simulink model "allmodes"  (Simulink 7.4)
settings: Solver=ode23tb  StartTime=0.0  StopTime=inf  MaxStep=1e-4  RelTol=1e-4
undefined symbols (not defined in the file): Ion, Lithium
libraries: powerlib x185, electricdrivelib x21, powerlib_extras x19, simulink x5
(part 4 of 7)

== system allmodes/vechicle units/vechicle-1 ==
  C1v1 : powerlib/Elements/Series RLC Branch  DialogController=POWERSYS.PowerSysDialog  PhysicalDomain=powersysdomain  SubClassName=unknown  LeftPortType=p1  RightPortType=p1  LConnTagsString=__new0  RConnTagsString=__new0  BranchType=C  Resistance=0.75  Inductance=1e-3  SetiL0=off  InitialCurrent=0  Capacitance=33e-5  Setx0=on  InitialVoltage=0  Measurements=Branch voltage and current
  Demux3 : Demux  Outputs=3
  Demux4 : Demux  Outputs=3
  IGBT20 : Subsystem
  IGBT21 : Subsystem
  L11v1 : powerlib/Elements/Series RLC Branch  DialogController=POWERSYS.PowerSysDialog  PhysicalDomain=powersysdomain  SubClassName=unknown  LeftPortType=p1  RightPortType=p1  LConnTagsString=__new0  RConnTagsString=__new0  BranchType=RL  Resistance=1e-3  Inductance=0.0033  SetiL0=off  InitialCurrent=0  Capacitance=1e-6  Setx0=off  InitialVoltage=0  Measurements=Branch voltage and current
  L22v1 : powerlib/Elements/Series RLC Branch  DialogController=POWERSYS.PowerSysDialog  PhysicalDomain=powersysdomain  SubClassName=unknown  LeftPortType=p1  RightPortType=p1  LConnTagsString=__new0  RConnTagsString=__new0  BranchType=RL  Resistance=1e-3  Inductance=1.2e-4  SetiL0=off  InitialCurrent=0  Capacitance=1e-6  Setx0=off  InitialVoltage=0  Measurements=Branch current
  Multimeter3 : powerlib/Measurements/Multimeter  SystemSampleTime=-1  PhasorSimulation=off  OutputType=Complex  sel=[5 58 59]  L=119  Gain=[1 1 1]  yselected={'Ub: vechicle units/vechicle-1/C1v1','Ib: vechicle units/vechicle-1/L11v1','Ib: vechicle units/vechicle-1/L22v1'};  PSBOutputType=1  PSBequivalent=0  AxesSetting=[0,0.1,-100,100]  Display=0  SavedBlockNames=-11
  v-1 : electricdrivelib/Extra Sources/Battery  DialogController=POWERSYS.PowerSysDialog  SystemSampleTime=-1  BatType=Lithium-Ion  ShowDetailedParameters=off  NomV=200  NomQ=30  SOC=10  PresetModel=on  MaxQ=30  FullV=232.7974  Dis_rate=13.0435  R=0.066667  Normal_OP=27.1304  expZone="[216.0772      1.473913]"  Dis_Char=off  current=[1.5 70]  Units=Ampere-hour  Batt_Tr=30
  +ve : PMIOPort  Port=1  Side=Left
  -ve : PMIOPort  Port=2  Side=Left
  tag scope: ISUIMv1=global, IbSUIMv1=global, Ibatv1=global, VbSUIMv1=global, VcSUIMv1=global, socv1=global
  wires:
  v-1/1 -> Demux4/1
  Demux4/1 -> [socv1]
  Demux4/2 -> [Ibatv1]
  Demux4/3 -> [VbSUIMv1]
  Multimeter3/1 -> Demux3/1
  Demux3/2 -> [ISUIMv1]
  Demux3/3 -> [IbSUIMv1]
  Demux3/1 -> [VcSUIMv1]
  connections:
  C1v1/LConn1 -- L22v1/LConn1 -- L11v1/RConn1
  -ve/RConn1 -- IGBT21/RConn2 -- v-1/LConn2 -- C1v1/RConn1
  IGBT20/RConn2 -- L11v1/LConn1 -- IGBT21/RConn1
  L22v1/RConn1 -- v-1/LConn1
  +ve/RConn1 -- IGBT20/RConn1

== system allmodes/vechicle units/vechicle-10 ==
  C1v10 : powerlib/Elements/Series RLC Branch  DialogController=POWERSYS.PowerSysDialog  PhysicalDomain=powersysdomain  SubClassName=unknown  LeftPortType=p1  RightPortType=p1  LConnTagsString=__new0  RConnTagsString=__new0  BranchType=C  Resistance=0.75  Inductance=1e-3  SetiL0=off  InitialCurrent=0  Capacitance=33e-6  Setx0=on  InitialVoltage=0  Measurements=Branch voltage and current
  Demux3 : Demux  Outputs=3
  Demux4 : Demux  Outputs=3
  IGBT20 : Subsystem
  IGBT21 : Subsystem
  L11v10 : powerlib/Elements/Series RLC Branch  DialogController=POWERSYS.PowerSysDialog  PhysicalDomain=powersysdomain  SubClassName=unknown  LeftPortType=p1  RightPortType=p1  LConnTagsString=__new0  RConnTagsString=__new0  BranchType=RL  Resistance=1e-3  Inductance=0.0033  SetiL0=off  InitialCurrent=0  Capacitance=1e-6  Setx0=off  InitialVoltage=0  Measurements=Branch voltage and current
  L22v10 : powerlib/Elements/Series RLC Branch  DialogController=POWERSYS.PowerSysDialog  PhysicalDomain=powersysdomain  SubClassName=unknown  LeftPortType=p1  RightPortType=p1  LConnTagsString=__new0  RConnTagsString=__new0  BranchType=RL  Resistance=0.001  Inductance=1.2e-4  SetiL0=off  InitialCurrent=0  Capacitance=1e-6  Setx0=off  InitialVoltage=0  Measurements=Branch current
  Multimeter3 : powerlib/Measurements/Multimeter  SystemSampleTime=-1  PhasorSimulation=off  OutputType=Complex  sel=[7 61 62]  L=119  Gain=[1 1 1]  yselected={'Ub: vechicle units/vechicle-10/C1v10','Ib: vechicle units/vechicle-10/L11v10','Ib: vechicle units/vechicle-10/L22v10'};  PSBOutputType=1  PSBequivalent=0  AxesSetting=[0,0.1,-100,100]  Display=0  SavedBlockNames=-11
  v-10 : electricdrivelib/Extra Sources/Battery  DialogController=POWERSYS.PowerSysDialog  SystemSampleTime=-1  BatType=Lithium-Ion  ShowDetailedParameters=off  NomV=200  NomQ=30  SOC=50  PresetModel=on  MaxQ=30  FullV=232.7974  Dis_rate=13.0435  R=0.066667  Normal_OP=27.1304  expZone="[216.0772      1.473913]"  Dis_Char=off  current=[1.5 70]  Units=Ampere-hour  Batt_Tr=30
  +ve : PMIOPort  Port=1  Side=Left
  -ve : PMIOPort  Port=2  Side=Left
  tag scope: ISUIMv10=global, IbSUIMv10=global, Ibatv10=global, VbSUIMv10=global, VcSUIMv10=global, socv10=global
  wires:
  Demux3/1 -> [VcSUIMv10]
  Demux3/3 -> [IbSUIMv10]
  Demux3/2 -> [ISUIMv10]
  Multimeter3/1 -> Demux3/1
  Demux4/3 -> [VbSUIMv10]
  Demux4/2 -> [Ibatv10]
  Demux4/1 -> [socv10]
  v-10/1 -> Demux4/1
  connections:
  +ve/RConn1 -- IGBT20/RConn1
  L22v10/RConn1 -- v-10/LConn1
  IGBT21/RConn1 -- IGBT20/RConn2 -- L11v10/LConn1
  IGBT21/RConn2 -- -ve/RConn1 -- C1v10/RConn1 -- v-10/LConn2
  L11v10/RConn1 -- L22v10/LConn1 -- C1v10/LConn1

== system allmodes/vechicle units/vechicle-11 ==
  C1v11 : powerlib/Elements/Series RLC Branch  DialogController=POWERSYS.PowerSysDialog  PhysicalDomain=powersysdomain  SubClassName=unknown  LeftPortType=p1  RightPortType=p1  LConnTagsString=__new0  RConnTagsString=__new0  BranchType=C  Resistance=0.75  Inductance=1e-3  SetiL0=off  InitialCurrent=0  Capacitance=33e-6  Setx0=on  InitialVoltage=0  Measurements=Branch voltage and current
  Demux3 : Demux  Outputs=3
  Demux4 : Demux  Outputs=3
  IGBT20 : Subsystem
  IGBT21 : Subsystem
  L11v11 : powerlib/Elements/Series RLC Branch  DialogController=POWERSYS.PowerSysDialog  PhysicalDomain=powersysdomain  SubClassName=unknown  LeftPortType=p1  RightPortType=p1  LConnTagsString=__new0  RConnTagsString=__new0  BranchType=RL  Resistance=0.001  Inductance=0.0033  SetiL0=off  InitialCurrent=0  Capacitance=1e-6  Setx0=off  InitialVoltage=0  Measurements=Branch voltage and current
  L22v11 : powerlib/Elements/Series RLC Branch  DialogController=POWERSYS.PowerSysDialog  PhysicalDomain=powersysdomain  SubClassName=unknown  LeftPortType=p1  RightPortType=p1  LConnTagsString=__new0  RConnTagsString=__new0  BranchType=RL  Resistance=0.001  Inductance=1.2e-4  SetiL0=off  InitialCurrent=0  Capacitance=1e-6  Setx0=off  InitialVoltage=0  Measurements=Branch current
  Multimeter3 : powerlib/Measurements/Multimeter  SystemSampleTime=-1  PhasorSimulation=off  OutputType=Complex  sel=[9 64 65]  L=119  Gain=[1 1 1]  yselected={'Ub: vechicle units/vechicle-11/C1v11','Ib: vechicle units/vechicle-11/L11v11','Ib: vechicle units/vechicle-11/L22v11'};  PSBOutputType=1  PSBequivalent=0  AxesSetting=[0,0.1,-100,100]  Display=0  SavedBlockNames=-11
  v-11 : electricdrivelib/Extra Sources/Battery  DialogController=POWERSYS.PowerSysDialog  SystemSampleTime=-1  BatType=Lithium-Ion  ShowDetailedParameters=off  NomV=200  NomQ=30  SOC=50  PresetModel=on  MaxQ=30  FullV=232.7974  Dis_rate=13.0435  R=0.066667  Normal_OP=27.1304  expZone="[216.0772      1.473913]"  Dis_Char=off  current=[1.5 70]  Units=Ampere-hour  Batt_Tr=30
  +ve : PMIOPort  Port=1  Side=Left
  -ve : PMIOPort  Port=2  Side=Left
  tag scope: ISUIMv11=global, IbSUIMv11=global, Ibatv11=global, VbSUIMv11=global, VcSUIMv11=global, socv11=global
  wires:
  v-11/1 -> Demux4/1
  Demux4/1 -> [socv11]
  Demux4/2 -> [Ibatv11]
  Demux4/3 -> [VbSUIMv11]
  Multimeter3/1 -> Demux3/1
  Demux3/2 -> [ISUIMv11]
  Demux3/3 -> [IbSUIMv11]
  Demux3/1 -> [VcSUIMv11]
  connections:
  C1v11/LConn1 -- L22v11/LConn1 -- L11v11/RConn1
  v-11/LConn2 -- C1v11/RConn1 -- -ve/RConn1 -- IGBT21/RConn2
  L11v11/LConn1 -- IGBT20/RConn2 -- IGBT21/RConn1
  L22v11/RConn1 -- v-11/LConn1
  +ve/RConn1 -- IGBT20/RConn1

== system allmodes/vechicle units/vechicle-12 ==
  C1v12 : powerlib/Elements/Series RLC Branch  DialogController=POWERSYS.PowerSysDialog  PhysicalDomain=powersysdomain  SubClassName=unknown  LeftPortType=p1  RightPortType=p1  LConnTagsString=__new0  RConnTagsString=__new0  BranchType=C  Resistance=0.75  Inductance=1e-3  SetiL0=off  InitialCurrent=0  Capacitance=33e-6  Setx0=on  InitialVoltage=0  Measurements=Branch voltage and current
  Demux3 : Demux  Outputs=3
  Demux4 : Demux  Outputs=3
  IGBT20 : Subsystem
  IGBT21 : Subsystem
  L11v12 : powerlib/Elements/Series RLC Branch  DialogController=POWERSYS.PowerSysDialog  PhysicalDomain=powersysdomain  SubClassName=unknown  LeftPortType=p1  RightPortType=p1  LConnTagsString=__new0  RConnTagsString=__new0  BranchType=RL  Resistance=0.001  Inductance=0.0033  SetiL0=off  InitialCurrent=0  Capacitance=1e-6  Setx0=off  InitialVoltage=0  Measurements=Branch voltage and current
  L22v12 : powerlib/Elements/Series RLC Branch  DialogController=POWERSYS.PowerSysDialog  PhysicalDomain=powersysdomain  SubClassName=unknown  LeftPortType=p1  RightPortType=p1  LConnTagsString=__new0  RConnTagsString=__new0  BranchType=RL  Resistance=0.001  Inductance=1.2e-4  SetiL0=off  InitialCurrent=0  Capacitance=1e-6  Setx0=off  InitialVoltage=0  Measurements=Branch current
  Multimeter3 : powerlib/Measurements/Multimeter  SystemSampleTime=-1  PhasorSimulation=off  OutputType=Complex  sel=[11 67 68]  L=119  Gain=[1 1 1]  yselected={'Ub: vechicle units/vechicle-12/C1v12','Ib: vechicle units/vechicle-12/L11v12','Ib: vechicle units/vechicle-12/L22v12'};  PSBOutputType=1  PSBequivalent=0  AxesSetting=[0,0.1,-100,100]  Display=0  SavedBlockNames=-11
  v-12 : electricdrivelib/Extra Sources/Battery  DialogController=POWERSYS.PowerSysDialog  SystemSampleTime=-1  BatType=Lithium-Ion  ShowDetailedParameters=off  NomV=200  NomQ=30  SOC=50  PresetModel=on  MaxQ=30  FullV=232.7974  Dis_rate=13.0435  R=0.066667  Normal_OP=27.1304  expZone="[216.0772      1.473913]"  Dis_Char=off  current=[1.5 70]  Units=Ampere-hour  Batt_Tr=30
  +ve : PMIOPort  Port=1  Side=Left
  -ve : PMIOPort  Port=2  Side=Left
  tag scope: ISUIMv12=global, IbSUIMv12=global, Ibatv12=global, VbSUIMv12=global, VcSUIMv12=global, socv12=global
  wires:
  Demux3/1 -> [VcSUIMv12]
  Demux3/3 -> [IbSUIMv12]
  Demux3/2 -> [ISUIMv12]
  Multimeter3/1 -> Demux3/1
  Demux4/3 -> [VbSUIMv12]
  Demux4/2 -> [Ibatv12]
  Demux4/1 -> [socv12]
  v-12/1 -> Demux4/1
  connections:
  +ve/RConn1 -- IGBT20/RConn1
  L22v12/RConn1 -- v-12/LConn1
  IGBT21/RConn1 -- IGBT20/RConn2 -- L11v12/LConn1
  IGBT21/RConn2 -- -ve/RConn1 -- C1v12/RConn1 -- v-12/LConn2
  L11v12/RConn1 -- L22v12/LConn1 -- C1v12/LConn1

== system allmodes/vechicle units/vechicle-13 ==
  C1v13 : powerlib/Elements/Series RLC Branch  DialogController=POWERSYS.PowerSysDialog  PhysicalDomain=powersysdomain  SubClassName=unknown  LeftPortType=p1  RightPortType=p1  LConnTagsString=__new0  RConnTagsString=__new0  BranchType=C  Resistance=0.75  Inductance=1e-3  SetiL0=off  InitialCurrent=0  Capacitance=33e-6  Setx0=on  InitialVoltage=0  Measurements=Branch voltage and current
  Demux3 : Demux  Outputs=3
  Demux4 : Demux  Outputs=3
  IGBT20 : Subsystem
  IGBT21 : Subsystem
  L11v13 : powerlib/Elements/Series RLC Branch  DialogController=POWERSYS.PowerSysDialog  PhysicalDomain=powersysdomain  SubClassName=unknown  LeftPortType=p1  RightPortType=p1  LConnTagsString=__new0  RConnTagsString=__new0  BranchType=RL  Resistance=0.001  Inductance=0.0033  SetiL0=off  InitialCurrent=0  Capacitance=1e-6  Setx0=off  InitialVoltage=0  Measurements=Branch voltage and current
  L22v13 : powerlib/Elements/Series RLC Branch  DialogController=POWERSYS.PowerSysDialog  PhysicalDomain=powersysdomain  SubClassName=unknown  LeftPortType=p1  RightPortType=p1  LConnTagsString=__new0  RConnTagsString=__new0  BranchType=RL  Resistance=0.001  Inductance=1.2e-4  SetiL0=off  InitialCurrent=0  Capacitance=1e-6  Setx0=off  InitialVoltage=0  Measurements=Branch current
  Multimeter3 : powerlib/Measurements/Multimeter  SystemSampleTime=-1  PhasorSimulation=off  OutputType=Complex  sel=[13 70 71]  L=119  Gain=[1 1 1]  yselected={'Ub: vechicle units/vechicle-13/C1v13','Ib: vechicle units/vechicle-13/L11v13','Ib: vechicle units/vechicle-13/L22v13'};  PSBOutputType=1  PSBequivalent=0  AxesSetting=[0,0.1,-100,100]  Display=0  SavedBlockNames=-11
  v-13 : electricdrivelib/Extra Sources/Battery  DialogController=POWERSYS.PowerSysDialog  SystemSampleTime=-1  BatType=Lithium-Ion  ShowDetailedParameters=off  NomV=200  NomQ=30  SOC=50  PresetModel=on  MaxQ=30  FullV=232.7974  Dis_rate=13.0435  R=0.066667  Normal_OP=27.1304  expZone="[216.0772      1.473913]"  Dis_Char=off  current=[1.5 70]  Units=Ampere-hour  Batt_Tr=30
  +ve : PMIOPort  Port=1  Side=Left
  -ve : PMIOPort  Port=2  Side=Left
  tag scope: ISUIMv13=global, IbSUIMv13=global, Ibatv13=global, VbSUIMv13=global, VcSUIMv13=global, socv13=global
  wires:
  v-13/1 -> Demux4/1
  Demux4/1 -> [socv13]
  Demux4/2 -> [Ibatv13]
  Demux4/3 -> [VbSUIMv13]
  Multimeter3/1 -> Demux3/1
  Demux3/2 -> [ISUIMv13]
  Demux3/3 -> [IbSUIMv13]
  Demux3/1 -> [VcSUIMv13]
  connections:
  C1v13/LConn1 -- L22v13/LConn1 -- L11v13/RConn1
  v-13/LConn2 -- C1v13/RConn1 -- -ve/RConn1 -- IGBT21/RConn2
  L11v13/LConn1 -- IGBT20/RConn2 -- IGBT21/RConn1
  L22v13/RConn1 -- v-13/LConn1
  +ve/RConn1 -- IGBT20/RConn1

== system allmodes/vechicle units/vechicle-14 ==
  C1v14 : powerlib/Elements/Series RLC Branch  DialogController=POWERSYS.PowerSysDialog  PhysicalDomain=powersysdomain  SubClassName=unknown  LeftPortType=p1  RightPortType=p1  LConnTagsString=__new0  RConnTagsString=__new0  BranchType=C  Resistance=0.75  Inductance=1e-3  SetiL0=off  InitialCurrent=0  Capacitance=33e-6  Setx0=on  InitialVoltage=0  Measurements=Branch voltage and current
  Demux3 : Demux  Outputs=3
  Demux4 : Demux  Outputs=3
  IGBT20 : Subsystem
  IGBT21 : Subsystem
  L11v14 : powerlib/Elements/Series RLC Branch  DialogController=POWERSYS.PowerSysDialog  PhysicalDomain=powersysdomain  SubClassName=unknown  LeftPortType=p1  RightPortType=p1  LConnTagsString=__new0  RConnTagsString=__new0  BranchType=RL  Resistance=0.001  Inductance=0.0033  SetiL0=off  InitialCurrent=0  Capacitance=1e-6  Setx0=off  InitialVoltage=0  Measurements=Branch voltage and current
  L22v14 : powerlib/Elements/Series RLC Branch  DialogController=POWERSYS.PowerSysDialog  PhysicalDomain=powersysdomain  SubClassName=unknown  LeftPortType=p1  RightPortType=p1  LConnTagsString=__new0  RConnTagsString=__new0  BranchType=RL  Resistance=0.001  Inductance=1.2e-4  SetiL0=off  InitialCurrent=0  Capacitance=1e-6  Setx0=off  InitialVoltage=0  Measurements=Branch current
  Multimeter3 : powerlib/Measurements/Multimeter  SystemSampleTime=-1  PhasorSimulation=off  OutputType=Complex  sel=[15 73 74]  L=119  Gain=[1 1 1]  yselected={'Ub: vechicle units/vechicle-14/C1v14','Ib: vechicle units/vechicle-14/L11v14','Ib: vechicle units/vechicle-14/L22v14'};  PSBOutputType=1  PSBequivalent=0  AxesSetting=[0,0.1,-100,100]  Display=0  SavedBlockNames=-11
  v-14 : electricdrivelib/Extra Sources/Battery  DialogController=POWERSYS.PowerSysDialog  SystemSampleTime=-1  BatType=Lithium-Ion  ShowDetailedParameters=off  NomV=200  NomQ=30  SOC=50  PresetModel=on  MaxQ=30  FullV=232.7974  Dis_rate=13.0435  R=0.066667  Normal_OP=27.1304  expZone="[216.0772      1.473913]"  Dis_Char=off  current=[1.5 70]  Units=Ampere-hour  Batt_Tr=30
  +ve : PMIOPort  Port=1  Side=Left
  -ve : PMIOPort  Port=2  Side=Left
  tag scope: ISUIMv14=global, IbSUIMv14=global, Ibatv14=global, VbSUIMv14=global, VcSUIMv14=global, socv14=global
  wires:
  Demux3/1 -> [VcSUIMv14]
  Demux3/3 -> [IbSUIMv14]
  Demux3/2 -> [ISUIMv14]
  Multimeter3/1 -> Demux3/1
  Demux4/3 -> [VbSUIMv14]
  Demux4/2 -> [Ibatv14]
  Demux4/1 -> [socv14]
  v-14/1 -> Demux4/1
  connections:
  +ve/RConn1 -- IGBT20/RConn1
  L22v14/RConn1 -- v-14/LConn1
  IGBT21/RConn1 -- IGBT20/RConn2 -- L11v14/LConn1
  IGBT21/RConn2 -- -ve/RConn1 -- C1v14/RConn1 -- v-14/LConn2
  L11v14/RConn1 -- L22v14/LConn1 -- C1v14/LConn1

== system allmodes/vechicle units/vechicle-15 ==
  C1v15 : powerlib/Elements/Series RLC Branch  DialogController=POWERSYS.PowerSysDialog  PhysicalDomain=powersysdomain  SubClassName=unknown  LeftPortType=p1  RightPortType=p1  LConnTagsString=__new0  RConnTagsString=__new0  BranchType=C  Resistance=0.75  Inductance=1e-3  SetiL0=off  InitialCurrent=0  Capacitance=33e-6  Setx0=on  InitialVoltage=0  Measurements=Branch voltage and current
  Demux3 : Demux  Outputs=3
  Demux4 : Demux  Outputs=3
  IGBT20 : Subsystem
  IGBT21 : Subsystem
  L11v15 : powerlib/Elements/Series RLC Branch  DialogController=POWERSYS.PowerSysDialog  PhysicalDomain=powersysdomain  SubClassName=unknown  LeftPortType=p1  RightPortType=p1  LConnTagsString=__new0  RConnTagsString=__new0  BranchType=RL  Resistance=0.001  Inductance=0.0033  SetiL0=off  InitialCurrent=0  Capacitance=1e-6  Setx0=off  InitialVoltage=0  Measurements=Branch voltage and current
  L22v15 : powerlib/Elements/Series RLC Branch  DialogController=POWERSYS.PowerSysDialog  PhysicalDomain=powersysdomain  SubClassName=unknown  LeftPortType=p1  RightPortType=p1  LConnTagsString=__new0  RConnTagsString=__new0  BranchType=RL  Resistance=0.001  Inductance=1.21e-4  SetiL0=off  InitialCurrent=0  Capacitance=1e-6  Setx0=off  InitialVoltage=0  Measurements=Branch current
  Multimeter3 : powerlib/Measurements/Multimeter  SystemSampleTime=-1  PhasorSimulation=off  OutputType=Complex  sel=[17 76 77]  L=119  Gain=[1 1 1]  yselected={'Ub: vechicle units/vechicle-15/C1v15','Ib: vechicle units/vechicle-15/L11v15','Ib: vechicle units/vechicle-15/L22v15'};  PSBOutputType=1  PSBequivalent=0  AxesSetting=[0,0.1,-100,100]  Display=0  SavedBlockNames=-11
  v-15 : electricdrivelib/Extra Sources/Battery  DialogController=POWERSYS.PowerSysDialog  SystemSampleTime=-1  BatType=Lithium-Ion  ShowDetailedParameters=off  NomV=200  NomQ=30  SOC=50  PresetModel=on  MaxQ=30  FullV=232.7974  Dis_rate=13.0435  R=0.066667  Normal_OP=27.1304  expZone="[216.0772      1.473913]"  Dis_Char=off  current=[1.5 70]  Units=Ampere-hour  Batt_Tr=30
  +ve : PMIOPort  Port=1  Side=Left
  -ve : PMIOPort  Port=2  Side=Left
  tag scope: ISUIMv15=global, IbSUIMv15=global, Ibatv15=global, VbSUIMv15=global, VcSUIMv15=global, socv15=global
  wires:
  v-15/1 -> Demux4/1
  Demux4/1 -> [socv15]
  Demux4/2 -> [Ibatv15]
  Demux4/3 -> [VbSUIMv15]
  Multimeter3/1 -> Demux3/1
  Demux3/2 -> [ISUIMv15]
  Demux3/3 -> [IbSUIMv15]
  Demux3/1 -> [VcSUIMv15]
  connections:
  C1v15/LConn1 -- L22v15/LConn1 -- L11v15/RConn1
  v-15/LConn2 -- C1v15/RConn1 -- -ve/RConn1 -- IGBT21/RConn2
  L11v15/LConn1 -- IGBT20/RConn2 -- IGBT21/RConn1
  L22v15/RConn1 -- v-15/LConn1
  +ve/RConn1 -- IGBT20/RConn1

== system allmodes/vechicle units/vechicle-16 ==
  C1v16 : powerlib/Elements/Series RLC Branch  DialogController=POWERSYS.PowerSysDialog  PhysicalDomain=powersysdomain  SubClassName=unknown  LeftPortType=p1  RightPortType=p1  LConnTagsString=__new0  RConnTagsString=__new0  BranchType=C  Resistance=0.75  Inductance=1e-3  SetiL0=off  InitialCurrent=0  Capacitance=33e-6  Setx0=on  InitialVoltage=0  Measurements=Branch voltage and current
  Demux3 : Demux  Outputs=3
  Demux4 : Demux  Outputs=3
  IGBT20 : Subsystem
  IGBT21 : Subsystem
  L11v16 : powerlib/Elements/Series RLC Branch  DialogController=POWERSYS.PowerSysDialog  PhysicalDomain=powersysdomain  SubClassName=unknown  LeftPortType=p1  RightPortType=p1  LConnTagsString=__new0  RConnTagsString=__new0  BranchType=RL  Resistance=0.001  Inductance=0.0033  SetiL0=off  InitialCurrent=0  Capacitance=1e-6  Setx0=off  InitialVoltage=0  Measurements=Branch voltage and current
  L22v16 : powerlib/Elements/Series RLC Branch  DialogController=POWERSYS.PowerSysDialog  PhysicalDomain=powersysdomain  SubClassName=unknown  LeftPortType=p1  RightPortType=p1  LConnTagsString=__new0  RConnTagsString=__new0  BranchType=RL  Resistance=0.001  Inductance=1.2e-4  SetiL0=off  InitialCurrent=0  Capacitance=1e-6  Setx0=off  InitialVoltage=0  Measurements=Branch current
  Multimeter3 : powerlib/Measurements/Multimeter  SystemSampleTime=-1  PhasorSimulation=off  OutputType=Complex  sel=[19 79 80]  L=119  Gain=[1 1 1]  yselected={'Ub: vechicle units/vechicle-16/C1v16','Ib: vechicle units/vechicle-16/L11v16','Ib: vechicle units/vechicle-16/L22v16'};  PSBOutputType=1  PSBequivalent=0  AxesSetting=[0,0.1,-100,100]  Display=0  SavedBlockNames=-11
  v-16 : electricdrivelib/Extra Sources/Battery  DialogController=POWERSYS.PowerSysDialog  SystemSampleTime=-1  BatType=Lithium-Ion  ShowDetailedParameters=off  NomV=200  NomQ=30  SOC=50  PresetModel=on  MaxQ=30  FullV=232.7974  Dis_rate=13.0435  R=0.066667  Normal_OP=27.1304  expZone="[216.0772      1.473913]"  Dis_Char=off  current=[1.5 70]  Units=Ampere-hour  Batt_Tr=30
  +ve : PMIOPort  Port=1  Side=Left
  -ve : PMIOPort  Port=2  Side=Left
  tag scope: ISUIMv16=global, IbSUIMv16=global, Ibatv16=global, VbSUIMv16=global, VcSUIMv16=global, socv16=global
  wires:
  Demux3/1 -> [VcSUIMv16]
  Demux3/3 -> [IbSUIMv16]
  Demux3/2 -> [ISUIMv16]
  Multimeter3/1 -> Demux3/1
  Demux4/3 -> [VbSUIMv16]
  Demux4/2 -> [Ibatv16]
  Demux4/1 -> [socv16]
  v-16/1 -> Demux4/1
  connections:
  +ve/RConn1 -- IGBT20/RConn1
  L22v16/RConn1 -- v-16/LConn1
  IGBT21/RConn1 -- IGBT20/RConn2 -- L11v16/LConn1
  IGBT21/RConn2 -- -ve/RConn1 -- C1v16/RConn1 -- v-16/LConn2
  L11v16/RConn1 -- L22v16/LConn1 -- C1v16/LConn1

== system allmodes/vechicle units/vechicle-17 ==
  C1v17 : powerlib/Elements/Series RLC Branch  DialogController=POWERSYS.PowerSysDialog  PhysicalDomain=powersysdomain  SubClassName=unknown  LeftPortType=p1  RightPortType=p1  LConnTagsString=__new0  RConnTagsString=__new0  BranchType=C  Resistance=0.75  Inductance=1e-3  SetiL0=off  InitialCurrent=0  Capacitance=33e-6  Setx0=on  InitialVoltage=0  Measurements=Branch voltage and current
  Demux3 : Demux  Outputs=3
  Demux4 : Demux  Outputs=3
  IGBT20 : Subsystem
  IGBT21 : Subsystem
  L11v17 : powerlib/Elements/Series RLC Branch  DialogController=POWERSYS.PowerSysDialog  PhysicalDomain=powersysdomain  SubClassName=unknown  LeftPortType=p1  RightPortType=p1  LConnTagsString=__new0  RConnTagsString=__new0  BranchType=RL  Resistance=0.001  Inductance=0.0033  SetiL0=off  InitialCurrent=0  Capacitance=1e-6  Setx0=off  InitialVoltage=0  Measurements=Branch voltage and current
  L22v17 : powerlib/Elements/Series RLC Branch  DialogController=POWERSYS.PowerSysDialog  PhysicalDomain=powersysdomain  SubClassName=unknown  LeftPortType=p1  RightPortType=p1  LConnTagsString=__new0  RConnTagsString=__new0  BranchType=RL  Resistance=0.001  Inductance=1.2e-4  SetiL0=off  InitialCurrent=0  Capacitance=1e-6  Setx0=off  InitialVoltage=0  Measurements=Branch current
  Multimeter3 : powerlib/Measurements/Multimeter  SystemSampleTime=-1  PhasorSimulation=off  OutputType=Complex  sel=[21 82 83]  L=119  Gain=[1 1 1]  yselected={'Ub: vechicle units/vechicle-17/C1v17','Ib: vechicle units/vechicle-17/L11v17','Ib: vechicle units/vechicle-17/L22v17'};  PSBOutputType=1  PSBequivalent=0  AxesSetting=[0,0.1,-100,100]  Display=0  SavedBlockNames=-11
  v-17 : electricdrivelib/Extra Sources/Battery  DialogController=POWERSYS.PowerSysDialog  SystemSampleTime=-1  BatType=Lithium-Ion  ShowDetailedParameters=off  NomV=200  NomQ=30  SOC=50  PresetModel=on  MaxQ=30  FullV=232.7974  Dis_rate=13.0435  R=0.066667  Normal_OP=27.1304  expZone="[216.0772      1.473913]"  Dis_Char=off  current=[1.5 70]  Units=Ampere-hour  Batt_Tr=30
  +ve : PMIOPort  Port=1  Side=Left
  -ve : PMIOPort  Port=2  Side=Left
  tag scope: ISUIMv17=global, IbSUIMv17=global, Ibatv17=global, VbSUIMv17=global, VcSUIMv17=global, socv17=global
  wires:
  v-17/1 -> Demux4/1
  Demux4/1 -> [socv17]
  Demux4/2 -> [Ibatv17]
  Demux4/3 -> [VbSUIMv17]
  Multimeter3/1 -> Demux3/1
  Demux3/2 -> [ISUIMv17]
  Demux3/3 -> [IbSUIMv17]
  Demux3/1 -> [VcSUIMv17]
  connections:
  C1v17/LConn1 -- L22v17/LConn1 -- L11v17/RConn1
  v-17/LConn2 -- C1v17/RConn1 -- -ve/RConn1 -- IGBT21/RConn2
  L11v17/LConn1 -- IGBT20/RConn2 -- IGBT21/RConn1
  L22v17/RConn1 -- v-17/LConn1
  +ve/RConn1 -- IGBT20/RConn1

== system allmodes/vechicle units/vechicle-18 ==
  C1v18 : powerlib/Elements/Series RLC Branch  DialogController=POWERSYS.PowerSysDialog  PhysicalDomain=powersysdomain  SubClassName=unknown  LeftPortType=p1  RightPortType=p1  LConnTagsString=__new0  RConnTagsString=__new0  BranchType=C  Resistance=0.75  Inductance=1e-3  SetiL0=off  InitialCurrent=0  Capacitance=33e-6  Setx0=on  InitialVoltage=0  Measurements=Branch voltage and current
  Demux3 : Demux  Outputs=3
  Demux4 : Demux  Outputs=3
  IGBT20 : Subsystem
  IGBT21 : Subsystem
  L11v18 : powerlib/Elements/Series RLC Branch  DialogController=POWERSYS.PowerSysDialog  PhysicalDomain=powersysdomain  SubClassName=unknown  LeftPortType=p1  RightPortType=p1  LConnTagsString=__new0  RConnTagsString=__new0  BranchType=RL  Resistance=0.001  Inductance=0.0033  SetiL0=off  InitialCurrent=0  Capacitance=1e-6  Setx0=off  InitialVoltage=0  Measurements=Branch voltage and current
  L22v18 : powerlib/Elements/Series RLC Branch  DialogController=POWERSYS.PowerSysDialog  PhysicalDomain=powersysdomain  SubClassName=unknown  LeftPortType=p1  RightPortType=p1  LConnTagsString=__new0  RConnTagsString=__new0  BranchType=RL  Resistance=0.001  Inductance=1.2e-4  SetiL0=off  InitialCurrent=0  Capacitance=1e-6  Setx0=off  InitialVoltage=0  Measurements=Branch current
  Multimeter3 : powerlib/Measurements/Multimeter  SystemSampleTime=-1  PhasorSimulation=off  OutputType=Complex  sel=[23 85 86]  L=119  Gain=[1 1 1]  yselected={'Ub: vechicle units/vechicle-18/C1v18','Ib: vechicle units/vechicle-18/L11v18','Ib: vechicle units/vechicle-18/L22v18'};  PSBOutputType=1  PSBequivalent=0  AxesSetting=[0,0.1,-100,100]  Display=0  SavedBlockNames=-11
  v-18 : electricdrivelib/Extra Sources/Battery  DialogController=POWERSYS.PowerSysDialog  SystemSampleTime=-1  BatType=Lithium-Ion  ShowDetailedParameters=off  NomV=200  NomQ=30  SOC=50  PresetModel=on  MaxQ=30  FullV=232.7974  Dis_rate=13.0435  R=0.066667  Normal_OP=27.1304  expZone="[216.0772      1.473913]"  Dis_Char=off  current=[1.5 70]  Units=Ampere-hour  Batt_Tr=30
  +ve : PMIOPort  Port=1  Side=Left
  -ve : PMIOPort  Port=2  Side=Left
  tag scope: ISUIMv18=global, IbSUIMv18=global, Ibatv18=global, VbSUIMv18=global, VcSUIMv18=global, socv18=global
  wires:
  Demux3/1 -> [VcSUIMv18]
  Demux3/3 -> [IbSUIMv18]
  Demux3/2 -> [ISUIMv18]
  Multimeter3/1 -> Demux3/1
  Demux4/3 -> [VbSUIMv18]
  Demux4/2 -> [Ibatv18]
  Demux4/1 -> [socv18]
  v-18/1 -> Demux4/1
  connections:
  +ve/RConn1 -- IGBT20/RConn1
  L22v18/RConn1 -- v-18/LConn1
  IGBT21/RConn1 -- IGBT20/RConn2 -- L11v18/LConn1
  IGBT21/RConn2 -- -ve/RConn1 -- C1v18/RConn1 -- v-18/LConn2
  L11v18/RConn1 -- L22v18/LConn1 -- C1v18/LConn1

== system allmodes/vechicle units/vechicle-19 ==
  C1v19 : powerlib/Elements/Series RLC Branch  DialogController=POWERSYS.PowerSysDialog  PhysicalDomain=powersysdomain  SubClassName=unknown  LeftPortType=p1  RightPortType=p1  LConnTagsString=__new0  RConnTagsString=__new0  BranchType=C  Resistance=0.75  Inductance=1e-3  SetiL0=off  InitialCurrent=0  Capacitance=33e-6  Setx0=on  InitialVoltage=0  Measurements=Branch voltage and current
  Demux3 : Demux  Outputs=3
  Demux4 : Demux  Outputs=3
  IGBT20 : Subsystem
  IGBT21 : Subsystem
  L11v19 : powerlib/Elements/Series RLC Branch  DialogController=POWERSYS.PowerSysDialog  PhysicalDomain=powersysdomain  SubClassName=unknown  LeftPortType=p1  RightPortType=p1  LConnTagsString=__new0  RConnTagsString=__new0  BranchType=RL  Resistance=0.001  Inductance=0.0033  SetiL0=off  InitialCurrent=0  Capacitance=1e-6  Setx0=off  InitialVoltage=0  Measurements=Branch voltage and current
  L22v19 : powerlib/Elements/Series RLC Branch  DialogController=POWERSYS.PowerSysDialog  PhysicalDomain=powersysdomain  SubClassName=unknown  LeftPortType=p1  RightPortType=p1  LConnTagsString=__new0  RConnTagsString=__new0  BranchType=RL  Resistance=0.001  Inductance=1.2e-4  SetiL0=off  InitialCurrent=0  Capacitance=1e-6  Setx0=off  InitialVoltage=0  Measurements=Branch current
  Multimeter3 : powerlib/Measurements/Multimeter  SystemSampleTime=-1  PhasorSimulation=off  OutputType=Complex  sel=[25 88 89]  L=119  Gain=[1 1 1]  yselected={'Ub: vechicle units/vechicle-19/C1v19','Ib: vechicle units/vechicle-19/L11v19','Ib: vechicle units/vechicle-19/L22v19'};  PSBOutputType=1  PSBequivalent=0  AxesSetting=[0,0.1,-100,100]  Display=0  SavedBlockNames=-11
  v-19 : electricdrivelib/Extra Sources/Battery  DialogController=POWERSYS.PowerSysDialog  SystemSampleTime=-1  BatType=Lithium-Ion  ShowDetailedParameters=off  NomV=200  NomQ=30  SOC=50  PresetModel=on  MaxQ=30  FullV=232.7974  Dis_rate=13.0435  R=0.066667  Normal_OP=27.1304  expZone="[216.0772      1.473913]"  Dis_Char=off  current=[1.5 70]  Units=Ampere-hour  Batt_Tr=30
  +ve : PMIOPort  Port=1  Side=Left
  -ve : PMIOPort  Port=2  Side=Left
  tag scope: ISUIMv19=global, IbSUIMv19=global, Ibatv19=global, VbSUIMv19=global, VcSUIMv19=global, socv19=global
  wires:
  v-19/1 -> Demux4/1
  Demux4/1 -> [socv19]
  Demux4/2 -> [Ibatv19]
  Demux4/3 -> [VbSUIMv19]
  Multimeter3/1 -> Demux3/1
  Demux3/2 -> [ISUIMv19]
  Demux3/3 -> [IbSUIMv19]
  Demux3/1 -> [VcSUIMv19]
  connections:
  C1v19/LConn1 -- L22v19/LConn1 -- L11v19/RConn1
  v-19/LConn2 -- C1v19/RConn1 -- -ve/RConn1 -- IGBT21/RConn2
  L11v19/LConn1 -- IGBT20/RConn2 -- IGBT21/RConn1
  L22v19/RConn1 -- v-19/LConn1
  +ve/RConn1 -- IGBT20/RConn1

== system allmodes/vechicle units/vechicle-2 ==
  C1v2 : powerlib/Elements/Series RLC Branch  DialogController=POWERSYS.PowerSysDialog  PhysicalDomain=powersysdomain  SubClassName=unknown  LeftPortType=p1  RightPortType=p1  LConnTagsString=__new0  RConnTagsString=__new0  BranchType=C  Resistance=0.75  Inductance=1e-3  SetiL0=off  InitialCurrent=0  Capacitance=33e-6  Setx0=on  InitialVoltage=0  Measurements=Branch voltage and current
  Demux3 : Demux  Outputs=3
  Demux4 : Demux  Outputs=3
  IGBT20 : Subsystem
  IGBT21 : Subsystem
  L11v2 : powerlib/Elements/Series RLC Branch  DialogController=POWERSYS.PowerSysDialog  PhysicalDomain=powersysdomain  SubClassName=unknown  LeftPortType=p1  RightPortType=p1  LConnTagsString=__new0  RConnTagsString=__new0  BranchType=RL  Resistance=00.001  Inductance=0.0033  SetiL0=off  InitialCurrent=0  Capacitance=1e-6  Setx0=off  InitialVoltage=0  Measurements=Branch voltage and current
  L22v2 : powerlib/Elements/Series RLC Branch  DialogController=POWERSYS.PowerSysDialog  PhysicalDomain=powersysdomain  SubClassName=unknown  LeftPortType=p1  RightPortType=p1  LConnTagsString=__new0  RConnTagsString=__new0  BranchType=RL  Resistance=0.001  Inductance=1.2e-3  SetiL0=off  InitialCurrent=0  Capacitance=1e-6  Setx0=off  InitialVoltage=0  Measurements=Branch current
  Multimeter3 : powerlib/Measurements/Multimeter  SystemSampleTime=-1  PhasorSimulation=off  OutputType=Complex  sel=[27 91 92]  L=119  Gain=[1 1 1]  yselected={'Ub: vechicle units/vechicle-2/C1v2','Ib: vechicle units/vechicle-2/L11v2','Ib: vechicle units/vechicle-2/L22v2'};  PSBOutputType=1  PSBequivalent=0  AxesSetting=[0,0.1,-100,100]  Display=0  SavedBlockNames=-11
  v-2 : electricdrivelib/Extra Sources/Battery  DialogController=POWERSYS.PowerSysDialog  SystemSampleTime=-1  BatType=Lithium-Ion  ShowDetailedParameters=off  NomV=200  NomQ=30  SOC=50  PresetModel=on  MaxQ=30  FullV=232.7974  Dis_rate=13.0435  R=0.066667  Normal_OP=27.1304  expZone="[216.0772      1.473913]"  Dis_Char=off  current=[1.5 70]  Units=Ampere-hour  Batt_Tr=30
  +ve : PMIOPort  Port=1  Side=Left
  -ve : PMIOPort  Port=2  Side=Left
  tag scope: ISUIMv2=global, IbSUIMv2=global, Ibatv2=global, VbSUIMv2=global, VcSUIMv2=global, socv2=global
  wires:
  Demux3/1 -> [VcSUIMv2]
  Demux3/3 -> [IbSUIMv2]
  Demux3/2 -> [ISUIMv2]
  Multimeter3/1 -> Demux3/1
  Demux4/3 -> [VbSUIMv2]
  Demux4/2 -> [Ibatv2]
  Demux4/1 -> [socv2]
  v-2/1 -> Demux4/1
  connections:
  +ve/RConn1 -- IGBT20/RConn1
  L22v2/RConn1 -- v-2/LConn1
  IGBT21/RConn1 -- IGBT20/RConn2 -- L11v2/LConn1
  IGBT21/RConn2 -- -ve/RConn1 -- C1v2/RConn1 -- v-2/LConn2
  L11v2/RConn1 -- L22v2/LConn1 -- C1v2/LConn1

== system allmodes/vechicle units/vechicle-20 ==
  C1v20 : powerlib/Elements/Series RLC Branch  DialogController=POWERSYS.PowerSysDialog  PhysicalDomain=powersysdomain  SubClassName=unknown  LeftPortType=p1  RightPortType=p1  LConnTagsString=__new0  RConnTagsString=__new0  BranchType=C  Resistance=0.75  Inductance=1e-3  SetiL0=off  InitialCurrent=0  Capacitance=33e-6  Setx0=on  InitialVoltage=0  Measurements=Branch voltage and current
  Demux3 : Demux  Outputs=3
  Demux4 : Demux  Outputs=3
  IGBT20 : Subsystem
  IGBT21 : Subsystem
  L11v20 : powerlib/Elements/Series RLC Branch  DialogController=POWERSYS.PowerSysDialog  PhysicalDomain=powersysdomain  SubClassName=unknown  LeftPortType=p1  RightPortType=p1  LConnTagsString=__new0  RConnTagsString=__new0  BranchType=RL  Resistance=0.001  Inductance=0.0033  SetiL0=off  InitialCurrent=0  Capacitance=1e-6  Setx0=off  InitialVoltage=0  Measurements=Branch voltage and current
  L22v20 : powerlib/Elements/Series RLC Branch  DialogController=POWERSYS.PowerSysDialog  PhysicalDomain=powersysdomain  SubClassName=unknown  LeftPortType=p1  RightPortType=p1  LConnTagsString=__new0  RConnTagsString=__new0  BranchType=RL  Resistance=0.001  Inductance=1.2e-4  SetiL0=off  InitialCurrent=0  Capacitance=1e-6  Setx0=off  InitialVoltage=0  Measurements=Branch current
  Multimeter3 : powerlib/Measurements/Multimeter  SystemSampleTime=-1  PhasorSimulation=off  OutputType=Complex  sel=[29 94 95]  L=119  Gain=[1 1 1]  yselected={'Ub: vechicle units/vechicle-20/C1v20','Ib: vechicle units/vechicle-20/L11v20','Ib: vechicle units/vechicle-20/L22v20'};  PSBOutputType=1  PSBequivalent=0  AxesSetting=[0,0.1,-100,100]  Display=0  SavedBlockNames=-11
  v-20 : electricdrivelib/Extra Sources/Battery  DialogController=POWERSYS.PowerSysDialog  SystemSampleTime=-1  BatType=Lithium-Ion  ShowDetailedParameters=off  NomV=200  NomQ=30  SOC=50  PresetModel=on  MaxQ=30  FullV=232.7974  Dis_rate=13.0435  R=0.066667  Normal_OP=27.1304  expZone="[216.0772      1.473913]"  Dis_Char=off  current=[1.5 70]  Units=Ampere-hour  Batt_Tr=30
  +ve : PMIOPort  Port=1  Side=Left
  -ve : PMIOPort  Port=2  Side=Left
  tag scope: ISUIMv20=global, IbSUIMv20=global, Ibatv20=global, VbSUIMv20=global, VcSUIMv20=global, socv20=global
  wires:
  Demux3/1 -> [VcSUIMv20]
  Demux3/3 -> [IbSUIMv20]
  Demux3/2 -> [ISUIMv20]
  Multimeter3/1 -> Demux3/1
  Demux4/3 -> [VbSUIMv20]
  Demux4/2 -> [Ibatv20]
  Demux4/1 -> [socv20]
  v-20/1 -> Demux4/1
  connections:
  +ve/RConn1 -- IGBT20/RConn1
  L22v20/RConn1 -- v-20/LConn1
  IGBT21/RConn1 -- IGBT20/RConn2 -- L11v20/LConn1
  IGBT21/RConn2 -- -ve/RConn1 -- C1v20/RConn1 -- v-20/LConn2
  L11v20/RConn1 -- L22v20/LConn1 -- C1v20/LConn1

== system allmodes/vechicle units/vechicle-3 ==
  C1v3 : powerlib/Elements/Series RLC Branch  DialogController=POWERSYS.PowerSysDialog  PhysicalDomain=powersysdomain  SubClassName=unknown  LeftPortType=p1  RightPortType=p1  LConnTagsString=__new0  RConnTagsString=__new0  BranchType=C  Resistance=0.75  Inductance=1e-3  SetiL0=off  InitialCurrent=0  Capacitance=33e-6  Setx0=on  InitialVoltage=0  Measurements=Branch voltage and current
  Demux3 : Demux  Outputs=3
  Demux4 : Demux  Outputs=3
  IGBT20 : Subsystem
  IGBT21 : Subsystem
  L11v3 : powerlib/Elements/Series RLC Branch  DialogController=POWERSYS.PowerSysDialog  PhysicalDomain=powersysdomain  SubClassName=unknown  LeftPortType=p1  RightPortType=p1  LConnTagsString=__new0  RConnTagsString=__new0  BranchType=RL  Resistance=1e-3  Inductance=0.0033  SetiL0=off  InitialCurrent=0  Capacitance=1e-6  Setx0=off  InitialVoltage=0  Measurements=Branch voltage and current
  L22v3 : powerlib/Elements/Series RLC Branch  DialogController=POWERSYS.PowerSysDialog  PhysicalDomain=powersysdomain  SubClassName=unknown  LeftPortType=p1  RightPortType=p1  LConnTagsString=__new0  RConnTagsString=__new0  BranchType=RL  Resistance=1e-3  Inductance=1.2e-4  SetiL0=off  InitialCurrent=0  Capacitance=1e-6  Setx0=off  InitialVoltage=0  Measurements=Branch current
  Multimeter3 : powerlib/Measurements/Multimeter  SystemSampleTime=-1  PhasorSimulation=off  OutputType=Complex  sel=[31 97 98]  L=119  Gain=[1 1 1]  yselected={'Ub: vechicle units/vechicle-3/C1v3','Ib: vechicle units/vechicle-3/L11v3','Ib: vechicle units/vechicle-3/L22v3'};  PSBOutputType=1  PSBequivalent=0  AxesSetting=[0,0.1,-100,100]  Display=0  SavedBlockNames=-11
  v-3 : electricdrivelib/Extra Sources/Battery  DialogController=POWERSYS.PowerSysDialog  SystemSampleTime=-1  BatType=Lithium-Ion  ShowDetailedParameters=off  NomV=200  NomQ=30  SOC=50  PresetModel=on  MaxQ=30  FullV=232.7974  Dis_rate=13.0435  R=0.066667  Normal_OP=27.1304  expZone="[216.0772      1.473913]"  Dis_Char=off  current=[1.5 70]  Units=Ampere-hour  Batt_Tr=30
  +ve : PMIOPort  Port=1  Side=Left
  -ve : PMIOPort  Port=2  Side=Left
  tag scope: ISUIMv3=global, IbSUIMv3=global, Ibatv3=global, VbSUIMv3=global, VcSUIMv3=global, socv3=global
  wires:
  v-3/1 -> Demux4/1
  Demux4/1 -> [socv3]
  Demux4/2 -> [Ibatv3]
  Demux4/3 -> [VbSUIMv3]
  Multimeter3/1 -> Demux3/1
  Demux3/2 -> [ISUIMv3]
  Demux3/3 -> [IbSUIMv3]
  Demux3/1 -> [VcSUIMv3]
  connections:
  C1v3/LConn1 -- L22v3/LConn1 -- L11v3/RConn1
  v-3/LConn2 -- C1v3/RConn1 -- -ve/RConn1 -- IGBT21/RConn2
  L11v3/LConn1 -- IGBT20/RConn2 -- IGBT21/RConn1
  L22v3/RConn1 -- v-3/LConn1
  +ve/RConn1 -- IGBT20/RConn1

== system allmodes/vechicle units/vechicle-4 ==
  C1v4 : powerlib/Elements/Series RLC Branch  DialogController=POWERSYS.PowerSysDialog  PhysicalDomain=powersysdomain  SubClassName=unknown  LeftPortType=p1  RightPortType=p1  LConnTagsString=__new0  RConnTagsString=__new0  BranchType=C  Resistance=0.75  Inductance=1e-3  SetiL0=off  InitialCurrent=0  Capacitance=33e-6  Setx0=on  InitialVoltage=0  Measurements=Branch voltage and current
  Demux3 : Demux  Outputs=3
  Demux4 : Demux  Outputs=3
  IGBT20 : Subsystem
  IGBT21 : Subsystem
  L11v4 : powerlib/Elements/Series RLC Branch  DialogController=POWERSYS.PowerSysDialog  PhysicalDomain=powersysdomain  SubClassName=unknown  LeftPortType=p1  RightPortType=p1  LConnTagsString=__new0  RConnTagsString=__new0  BranchType=RL  Resistance=1e-3  Inductance=0.0033  SetiL0=off  InitialCurrent=0  Capacitance=1e-6  Setx0=off  InitialVoltage=0  Measurements=Branch voltage and current
  L22v4 : powerlib/Elements/Series RLC Branch  DialogController=POWERSYS.PowerSysDialog  PhysicalDomain=powersysdomain  SubClassName=unknown  LeftPortType=p1  RightPortType=p1  LConnTagsString=__new0  RConnTagsString=__new0  BranchType=RL  Resistance=1e-3  Inductance=1.2e-4  SetiL0=off  InitialCurrent=0  Capacitance=1e-6  Setx0=off  InitialVoltage=0  Measurements=Branch current
  Multimeter3 : powerlib/Measurements/Multimeter  SystemSampleTime=-1  PhasorSimulation=off  OutputType=Complex  sel=[33 100 101]  L=119  Gain=[1 1 1]  yselected={'Ub: vechicle units/vechicle-4/C1v4','Ib: vechicle units/vechicle-4/L11v4','Ib: vechicle units/vechicle-4/L22v4'};  PSBOutputType=1  PSBequivalent=0  AxesSetting=[0,0.1,-100,100]  Display=0  SavedBlockNames=-11
  v-4 : electricdrivelib/Extra Sources/Battery  DialogController=POWERSYS.PowerSysDialog  SystemSampleTime=-1  BatType=Lithium-Ion  ShowDetailedParameters=off  NomV=200  NomQ=30  SOC=50  PresetModel=on  MaxQ=30  FullV=232.7974  Dis_rate=13.0435  R=0.066667  Normal_OP=27.1304  expZone="[216.0772      1.473913]"  Dis_Char=off  current=[1.5 70]  Units=Ampere-hour  Batt_Tr=30
  +ve : PMIOPort  Port=1  Side=Left
  -ve : PMIOPort  Port=2  Side=Left
  tag scope: ISUIMv4=global, IbSUIMv4=global, Ibatv4=global, VbSUIMv4=global, VcSUIMv4=global, socv4=global
  wires:
  Demux3/1 -> [VcSUIMv4]
  Demux3/3 -> [IbSUIMv4]
  Demux3/2 -> [ISUIMv4]
  Multimeter3/1 -> Demux3/1
  Demux4/3 -> [VbSUIMv4]
  Demux4/2 -> [Ibatv4]
  Demux4/1 -> [socv4]
  v-4/1 -> Demux4/1
  connections:
  +ve/RConn1 -- IGBT20/RConn1
  L22v4/RConn1 -- v-4/LConn1
  IGBT21/RConn1 -- IGBT20/RConn2 -- L11v4/LConn1
  IGBT21/RConn2 -- -ve/RConn1 -- C1v4/RConn1 -- v-4/LConn2
  L11v4/RConn1 -- L22v4/LConn1 -- C1v4/LConn1

== system allmodes/vechicle units/vechicle-5 ==
  C1v5 : powerlib/Elements/Series RLC Branch  DialogController=POWERSYS.PowerSysDialog  PhysicalDomain=powersysdomain  SubClassName=unknown  LeftPortType=p1  RightPortType=p1  LConnTagsString=__new0  RConnTagsString=__new0  BranchType=C  Resistance=0.75  Inductance=1e-3  SetiL0=off  InitialCurrent=0  Capacitance=33e-6  Setx0=on  InitialVoltage=0  Measurements=Branch voltage and current
  Demux3 : Demux  Outputs=3
  Demux4 : Demux  Outputs=3
  IGBT20 : Subsystem
  IGBT21 : Subsystem
  L11v5 : powerlib/Elements/Series RLC Branch  DialogController=POWERSYS.PowerSysDialog  PhysicalDomain=powersysdomain  SubClassName=unknown  LeftPortType=p1  RightPortType=p1  LConnTagsString=__new0  RConnTagsString=__new0  BranchType=RL  Resistance=1e-3  Inductance=0.0033  SetiL0=off  InitialCurrent=0  Capacitance=1e-6  Setx0=off  InitialVoltage=0  Measurements=Branch voltage and current
  L22v5 : powerlib/Elements/Series RLC Branch  DialogController=POWERSYS.PowerSysDialog  PhysicalDomain=powersysdomain  SubClassName=unknown  LeftPortType=p1  RightPortType=p1  LConnTagsString=__new0  RConnTagsString=__new0  BranchType=RL  Resistance=0.001  Inductance=1.2e-4  SetiL0=off  InitialCurrent=0  Capacitance=1e-6  Setx0=off  InitialVoltage=0  Measurements=Branch current
  Multimeter3 : powerlib/Measurements/Multimeter  SystemSampleTime=-1  PhasorSimulation=off  OutputType=Complex  sel=[35 103 104]  L=119  Gain=[1 1 1]  yselected={'Ub: vechicle units/vechicle-5/C1v5','Ib: vechicle units/vechicle-5/L11v5','Ib: vechicle units/vechicle-5/L22v5'};  PSBOutputType=1  PSBequivalent=0  AxesSetting=[0,0.1,-100,100]  Display=0  SavedBlockNames=-11
  v-5 : electricdrivelib/Extra Sources/Battery  DialogController=POWERSYS.PowerSysDialog  SystemSampleTime=-1  BatType=Lithium-Ion  ShowDetailedParameters=off  NomV=200  NomQ=30  SOC=2  PresetModel=on  MaxQ=30  FullV=232.7974  Dis_rate=13.0435  R=0.066667  Normal_OP=27.1304  expZone="[216.0772      1.473913]"  Dis_Char=off  current=[1.5 70]  Units=Ampere-hour  Batt_Tr=30
  +ve : PMIOPort  Port=1  Side=Left
  -ve : PMIOPort  Port=2  Side=Left
  tag scope: ISUIMv5=global, IbSUIMv5=global, Ibatv5=global, VbSUIMv5=global, VcSUIMv5=global, socv5=global
  wires:
  v-5/1 -> Demux4/1
  Demux4/1 -> [socv5]
  Demux4/2 -> [Ibatv5]
  Demux4/3 -> [VbSUIMv5]
  Multimeter3/1 -> Demux3/1
  Demux3/2 -> [ISUIMv5]
  Demux3/3 -> [IbSUIMv5]
  Demux3/1 -> [VcSUIMv5]
  connections:
  C1v5/LConn1 -- L22v5/LConn1 -- L11v5/RConn1
  v-5/LConn2 -- C1v5/RConn1 -- -ve/RConn1 -- IGBT21/RConn2
  L11v5/LConn1 -- IGBT20/RConn2 -- IGBT21/RConn1
  L22v5/RConn1 -- v-5/LConn1
  +ve/RConn1 -- IGBT20/RConn1

== system allmodes/vechicle units/vechicle-6 ==
  C1v6 : powerlib/Elements/Series RLC Branch  DialogController=POWERSYS.PowerSysDialog  PhysicalDomain=powersysdomain  SubClassName=unknown  LeftPortType=p1  RightPortType=p1  LConnTagsString=__new0  RConnTagsString=__new0  BranchType=C  Resistance=0.75  Inductance=1e-3  SetiL0=off  InitialCurrent=0  Capacitance=33e-6  Setx0=on  InitialVoltage=0  Measurements=Branch voltage and current
  Demux3 : Demux  Outputs=3
  Demux4 : Demux  Outputs=3
  IGBT20 : Subsystem
  IGBT21 : Subsystem
  L11v6 : powerlib/Elements/Series RLC Branch  DialogController=POWERSYS.PowerSysDialog  PhysicalDomain=powersysdomain  SubClassName=unknown  LeftPortType=p1  RightPortType=p1  LConnTagsString=__new0  RConnTagsString=__new0  BranchType=RL  Resistance=0.001  Inductance=0.0033  SetiL0=off  InitialCurrent=0  Capacitance=1e-6  Setx0=off  InitialVoltage=0  Measurements=Branch voltage and current
  L22v6 : powerlib/Elements/Series RLC Branch  DialogController=POWERSYS.PowerSysDialog  PhysicalDomain=powersysdomain  SubClassName=unknown  LeftPortType=p1  RightPortType=p1  LConnTagsString=__new0  RConnTagsString=__new0  BranchType=RL  Resistance=0.001  Inductance=1.2e-4  SetiL0=off  InitialCurrent=0  Capacitance=1e-6  Setx0=off  InitialVoltage=0  Measurements=Branch current
  Multimeter3 : powerlib/Measurements/Multimeter  SystemSampleTime=-1  PhasorSimulation=off  OutputType=Complex  sel=[37 106 107]  L=119  Gain=[1 1 1]  yselected={'Ub: vechicle units/vechicle-6/C1v6','Ib: vechicle units/vechicle-6/L11v6','Ib: vechicle units/vechicle-6/L22v6'};  PSBOutputType=1  PSBequivalent=0  AxesSetting=[0,0.1,-100,100]  Display=0  SavedBlockNames=-11
  v-6 : electricdrivelib/Extra Sources/Battery  DialogController=POWERSYS.PowerSysDialog  SystemSampleTime=-1  BatType=Lithium-Ion  ShowDetailedParameters=off  NomV=200  NomQ=30  SOC=50  PresetModel=on  MaxQ=30  FullV=232.7974  Dis_rate=13.0435  R=0.066667  Normal_OP=27.1304  expZone="[216.0772      1.473913]"  Dis_Char=off  current=[1.5 70]  Units=Ampere-hour  Batt_Tr=30
  +ve : PMIOPort  Port=1  Side=Left
  -ve : PMIOPort  Port=2  Side=Left
  tag scope: ISUIMv6=global, IbSUIMv6=global, Ibatv6=global, VbSUIMv6=global, VcSUIMv6=global, socv6=global
  wires:
  Demux3/1 -> [VcSUIMv6]
  Demux3/3 -> [IbSUIMv6]
  Demux3/2 -> [ISUIMv6]
  Multimeter3/1 -> Demux3/1
  Demux4/3 -> [VbSUIMv6]
  Demux4/2 -> [Ibatv6]
  Demux4/1 -> [socv6]
  v-6/1 -> Demux4/1
  connections:
  +ve/RConn1 -- IGBT20/RConn1
  L22v6/RConn1 -- v-6/LConn1
  IGBT21/RConn1 -- IGBT20/RConn2 -- L11v6/LConn1
  IGBT21/RConn2 -- -ve/RConn1 -- C1v6/RConn1 -- v-6/LConn2
  L11v6/RConn1 -- L22v6/LConn1 -- C1v6/LConn1

== system allmodes/vechicle units/vechicle-7 ==
  C1v7 : powerlib/Elements/Series RLC Branch  DialogController=POWERSYS.PowerSysDialog  PhysicalDomain=powersysdomain  SubClassName=unknown  LeftPortType=p1  RightPortType=p1  LConnTagsString=__new0  RConnTagsString=__new0  BranchType=C  Resistance=0.75  Inductance=1e-3  SetiL0=off  InitialCurrent=0  Capacitance=33e-6  Setx0=on  InitialVoltage=0  Measurements=Branch voltage and current
  Demux3 : Demux  Outputs=3
  Demux4 : Demux  Outputs=3
  IGBT20 : Subsystem
  IGBT21 : Subsystem
  L11v7 : powerlib/Elements/Series RLC Branch  DialogController=POWERSYS.PowerSysDialog  PhysicalDomain=powersysdomain  SubClassName=unknown  LeftPortType=p1  RightPortType=p1  LConnTagsString=__new0  RConnTagsString=__new0  BranchType=RL  Resistance=0.0001  Inductance=0.00333  SetiL0=off  InitialCurrent=0  Capacitance=1e-6  Setx0=off  InitialVoltage=0  Measurements=Branch voltage and current
  L22v7 : powerlib/Elements/Series RLC Branch  DialogController=POWERSYS.PowerSysDialog  PhysicalDomain=powersysdomain  SubClassName=unknown  LeftPortType=p1  RightPortType=p1  LConnTagsString=__new0  RConnTagsString=__new0  BranchType=RL  Resistance=0.0001  Inductance=1.2e-4  SetiL0=off  InitialCurrent=0  Capacitance=1e-6  Setx0=off  InitialVoltage=0  Measurements=Branch current
  Multimeter3 : powerlib/Measurements/Multimeter  SystemSampleTime=-1  PhasorSimulation=off  OutputType=Complex  sel=[39 109 110]  L=119  Gain=[1 1 1]  yselected={'Ub: vechicle units/vechicle-7/C1v7','Ib: vechicle units/vechicle-7/L11v7','Ib: vechicle units/vechicle-7/L22v7'};  PSBOutputType=1  PSBequivalent=0  AxesSetting=[0,0.1,-100,100]  Display=0  SavedBlockNames=-11
  v-7 : electricdrivelib/Extra Sources/Battery  DialogController=POWERSYS.PowerSysDialog  SystemSampleTime=-1  BatType=Lithium-Ion  ShowDetailedParameters=off  NomV=200  NomQ=30  SOC=50  PresetModel=on  MaxQ=30  FullV=232.7974  Dis_rate=13.0435  R=0.066667  Normal_OP=27.1304  expZone="[216.0772      1.473913]"  Dis_Char=off  current=[1.5 70]  Units=Ampere-hour  Batt_Tr=30
  +ve : PMIOPort  Port=1  Side=Left
  -ve : PMIOPort  Port=2  Side=Left
  tag scope: ISUIMv7=global, IbSUIMv7=global, Ibatv7=global, VbSUIMv7=global, VcSUIMv7=global, socv7=global
  wires:
  v-7/1 -> Demux4/1
  Demux4/1 -> [socv7]
  Demux4/2 -> [Ibatv7]
  Demux4/3 -> [VbSUIMv7]
  Multimeter3/1 -> Demux3/1
  Demux3/2 -> [ISUIMv7]
  Demux3/3 -> [IbSUIMv7]
  Demux3/1 -> [VcSUIMv7]
  connections:
  L11v7/RConn1 -- C1v7/LConn1 -- L22v7/LConn1
  v-7/LConn2 -- C1v7/RConn1 -- -ve/RConn1 -- IGBT21/RConn2
  L11v7/LConn1 -- IGBT20/RConn2 -- IGBT21/RConn1
  L22v7/RConn1 -- v-7/LConn1
  +ve/RConn1 -- IGBT20/RConn1
